simulink model "b_2x_8a_r308d"  (Simulink 6.2)
settings: Solver=ode45  StartTime=0.0  StopTime=1030.0  RelTol=1e-3
undefined symbols (not defined in the file): ant_bits, BEE2_usr, blockCountBits, blockRowBits, cmult_4bit_em
libraries: xbsIndex_r3 x3300, xps_library x102, casper_library x97
(part 1 of 22)
settings Model: LastModifiedBy=manley
settings DebuggingCC: SolverPrmCheckMsg=warning

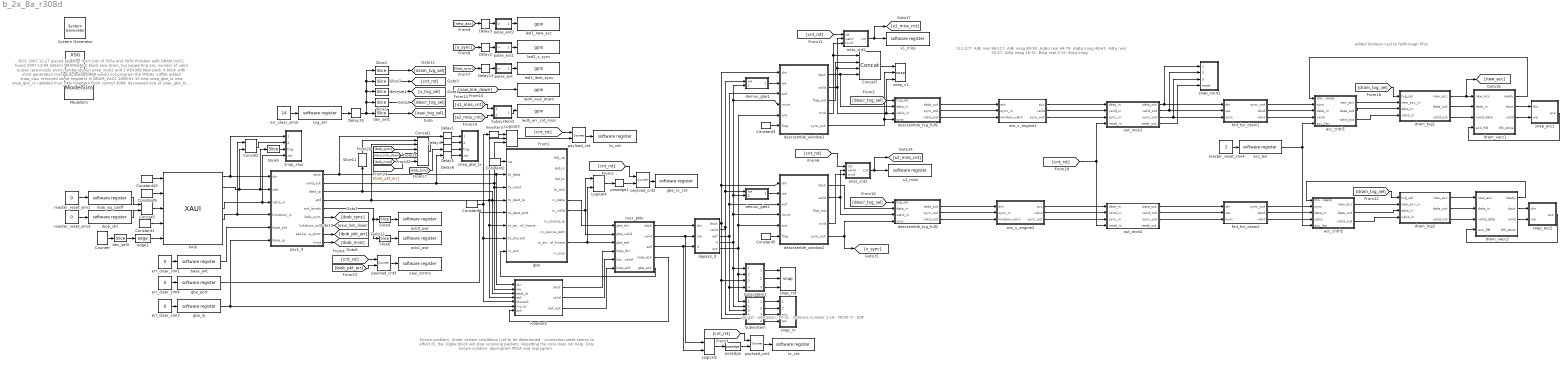
== system b_2x_8a_r308d ==
  note: 307c 2007-11-27
      | pieced together from bits of 307a and 307b
      | Problem with DRAM VACC found
      | 2007-12-04
      | Interim DRAM VACC block
      | new dram_tvg supporting any number of valid pulses (previously even numbers only)
      | snap_xout1 and 2
      | REV308
      | New pack_it block with mcnt generation moved to ibob
      |
      | BORPH would not program the FPGAs
      |
      | +308c
      | added snap_xaui
      | removed some registers in DRAM_VACC
      |
      | 2008-01-15
      | new snap_gbe_tx
      | new snap_gbe_rx
      | updated mux_pkts loopback flush control
      |
      | 308d:
      | decreased size of snap_gbe_tx, snap_gbe_rx blocks and snap_xout1 to ease routing
      | added dealy blocks to snap_gbe_tx
      | 22 Jan:
      | removed snap_gbe_rx, added snap_rx
      | 24 Jan:
      | replaced descramble onwards with version from rev307f
  note: Known problem:
      | Under certain conditions (yet to be determined - connection state seems to affect it),
      | the 10gbe block will stop receiving packets. Resetting the core does not help.
      | Only known solution: deprogram FPGA and reprogram.
  note: 112-127: AiBi real
      | 96-111: AiBi imag
      | 80-95: AqBq real
      | 64-79: AqBq imag
      | 48-63: AiBq real
      | 32-47: AiBq imag
      | 16-31: BiAq real
      | 0-15: BiAq imag
  note: added boolean cast to fallthrough fifos
  note: oob bit - allocation:
      | 17-31 - Antenna number
      | 1-16 - MCNT
      | 0 - EOF
  " System Generator" : xbsIndex_r3/ System Generator  Tag=genX  xilinxfamily=Virtex2P  part=xc2vp70  speed=-7  package=ff1704  synthesis_tool=XST  directory=./b_2x_8a_r308d/sysgen  testbench=off  simulink_period=1  sysclk_period=4.878  incr_netlist=off  trim_vbits=Everywhere in SubSystem  dbl_ovrd=According to Block Masks  core_generation=According to Block Masks  run_coregen=off  deprecated_control=off  eval_field=0
      settings: AttributesFormatString=System\nGenerator
  Concat1 : xbsIndex_r3/Concat  num_inputs=6  explicit_period=off  period=1  dbl_ovrd=off
  Concat2 : xbsIndex_r3/Concat  num_inputs=2  explicit_period=off  period=1  dbl_ovrd=off
  Concat3 : xbsIndex_r3/Concat  num_inputs=2  explicit_period=off  period=1  dbl_ovrd=off
  Concat7 : xbsIndex_r3/Concat  num_inputs=4  explicit_period=off  period=1  dbl_ovrd=off
  Constant1 : xbsIndex_r3/Constant  const=0  equ=P=C  arith_type=Unsigned  n_bits=64  bin_pt=0  opselect=C  inp2=PCIN>>17  opr=+  inp1=P  carry=CIN  iostate=0  explicit_period=on  period=1  dbl_ovrd=off
  Constant10 : xbsIndex_r3/Constant  const=1  equ=P=C  arith_type=Boolean  n_bits=1  bin_pt=0  opselect=C  inp2=PCIN>>17  opr=+  inp1=P  carry=CIN  iostate=0  explicit_period=on  period=1  dbl_ovrd=off
  Constant2 : xbsIndex_r3/Constant  const=0  equ=P=C  arith_type=Boolean  n_bits=1  bin_pt=0  opselect=C  inp2=PCIN>>17  opr=+  inp1=P  carry=CIN  iostate=0  explicit_period=on  period=1  dbl_ovrd=off
  Constant3 : xbsIndex_r3/Constant  const=0  equ=P=C  arith_type=Unsigned  n_bits=1  bin_pt=0  opselect=C  inp2=PCIN>>17  opr=+  inp1=P  carry=CIN  iostate=0  explicit_period=on  period=1  dbl_ovrd=off
  Constant5 : xbsIndex_r3/Constant  const=0  equ=P=C  arith_type=Unsigned  n_bits=1  bin_pt=0  opselect=C  inp2=PCIN>>17  opr=+  inp1=P  carry=CIN  iostate=0  explicit_period=on  period=1  dbl_ovrd=off
  Constant6 : xbsIndex_r3/Constant  const=0  equ=P=C  arith_type=Boolean  n_bits=16  bin_pt=0  opselect=C  inp2=PCIN>>17  opr=+  inp1=P  carry=CIN  iostate=0  explicit_period=on  period=1  dbl_ovrd=off
  Constant9 : xbsIndex_r3/Constant  const=0  equ=P=C  arith_type=Boolean  n_bits=1  bin_pt=0  opselect=C  inp2=PCIN>>17  opr=+  inp1=P  carry=CIN  iostate=0  explicit_period=on  period=1  dbl_ovrd=off
  Counter : xbsIndex_r3/Counter  cnt_type=Free Running  n_bits=4  bin_pt=0  arith_type=Unsigned  start_count=0  cnt_to=Inf  cnt_by_val=1  operation=Up  explicit_period=off  period=1  load_pin=off  rst=off  en=off  dbl_ovrd=off  show_param=off  use_rpm=on  gen_core=off
      settings: xl_area=[0, 0, 0, 0, 0, 0, 0]
  Delay{1,4..6,19} (5 alike) : xbsIndex_r3/Delay  latency=2  reg_retiming=on  explicit_period=off  period=1  en=off  accept_only_valid=off  init_zero=on  dbl_ovrd=off  show_param=off
      settings: xl_area=[0, 0, 0, 0, 0, 0, 0]
  Delay13 : xbsIndex_r3/Delay  latency=1  reg_retiming=on  explicit_period=off  period=1  en=off  accept_only_valid=off  init_zero=on  dbl_ovrd=off  show_param=off
      settings: xl_area=[0, 0, 0, 0, 0, 0, 0]
  Delay2 : xbsIndex_r3/Delay  latency=1  reg_retiming=on  explicit_period=off  period=1  en=off  accept_only_valid=off  init_zero=on  dbl_ovrd=off  show_param=off
      settings: xl_area=[0, 0, 0, 0, 0, 0, 0]
  Delay3 : xbsIndex_r3/Delay  latency=1  reg_retiming=on  explicit_period=off  period=1  en=off  accept_only_valid=off  init_zero=on  dbl_ovrd=off  show_param=off
      settings: xl_area=[0, 0, 0, 0, 0, 0, 0]
  Inverter3 : xbsIndex_r3/Inverter  latency=0  explicit_period=off  period=1  en=off  dbl_ovrd=off  show_param=off
      settings: xl_area=[0, 0, 0, 0, 0, 0, 0]
  Logical2 : xbsIndex_r3/Logical  logical_function=AND  inputs=2  precision=Full  arith_type=Unsigned  n_bits=8  bin_pt=2  align_bp=on  latency=0  explicit_period=on  period=1  en=off  dbl_ovrd=off  show_param=off
      settings: xl_area=[0, 0, 0, 0, 0, 0, 0]
  Logical3 : xbsIndex_r3/Logical  logical_function=AND  inputs=3  precision=Full  arith_type=Unsigned  n_bits=8  bin_pt=2  align_bp=on  latency=0  explicit_period=on  period=1  en=off  dbl_ovrd=off  show_param=off
      settings: xl_area=[0, 0, 0, 0, 0, 0, 0]
  Logical4 : xbsIndex_r3/Logical  logical_function=AND  inputs=2  precision=Full  arith_type=Unsigned  n_bits=8  bin_pt=2  align_bp=on  latency=0  explicit_period=on  period=1  en=off  dbl_ovrd=off  show_param=off
      settings: xl_area=[0, 0, 0, 0, 0, 0, 0]
  ModelSim : xbsIndex_r3/ModelSim  dir=./modelsim  waveform=on  leave_open=on  skip_compile=off  custom_scripts=off  startup_timeout=40
  Slice1 : xbsIndex_r3/Slice  mode=Lower Bit Location + Width  nbits=2  bit1=0  base1=MSB of Input  bit0=1  base0=LSB of Input  boolean_output=off  explicit_period=off  period=1  dbl_ovrd=off
  Slice11 : xbsIndex_r3/Slice  Orientation=up  mode=Lower Bit Location + Width  nbits=24  bit1=0  base1=MSB of Input  bit0=0  base0=LSB of Input  boolean_output=on  explicit_period=off  period=1  dbl_ovrd=off
  Slice2 : xbsIndex_r3/Slice  mode=Lower Bit Location + Width  nbits=6  bit1=0  base1=MSB of Input  bit0=9  base0=LSB of Input  boolean_output=off  explicit_period=off  period=1  dbl_ovrd=off
  Slice4 : xbsIndex_r3/Slice  mode=Lower Bit Location + Width  nbits=32  bit1=0  base1=MSB of Input  bit0=32  base0=LSB of Input  boolean_output=off  explicit_period=off  period=1  dbl_ovrd=off
  Slice6 : xbsIndex_r3/Slice  mode=Lower Bit Location + Width  nbits=32  bit1=0  base1=MSB of Input  bit0=0  base0=LSB of Input  boolean_output=off  explicit_period=off  period=1  dbl_ovrd=off
  Slice7 : xbsIndex_r3/Slice  mode=Lower Bit Location + Width  nbits=1  bit1=0  base1=MSB of Input  bit0=8  base0=LSB of Input  boolean_output=on  explicit_period=off  period=1  dbl_ovrd=off
  Slice9 : xbsIndex_r3/Slice  mode=Lower Bit Location + Width  nbits=1  bit1=0  base1=MSB of Input  bit0=1  base0=LSB of Input  boolean_output=on  explicit_period=off  period=1  dbl_ovrd=off
  Subsystem : Subsystem
  Subsystem1 : Subsystem
  Subsystem2 : Subsystem
  XAUI : xps_library/XAUI  Tag=xps:xaui  demux=1  port=BEE2_usr:0  show_param=off  pre_emph=3  swing=800
  XSG core config : xps_library/XSG core config  Tag=xps:xsg  hw_sys=BEE2_usr  ibob_linux=off  clk_src=sys_clk2x  gpio_clk_io_group=iBOB:sma  gpio_clk_bit_index=0  clk_rate=205  sample_period=1  synthesis_tool=XST  mpc_type=powerpc405
  acc_cntrl1 : Subsystem
  acc_cntrl2 : Subsystem
  acc_len : xps_library/software register  Tag=xps:sw_reg  io_dir=From Processor  arith_type=Unsigned  bitwidth=32  bin_pt=0  sample_period=1  gw_name=b_2x_8a_r308d_acc_len_user_data_out
  adc0_pwr : xps_library/software register  Tag=xps:sw_reg  io_dir=To Processor  arith_type=Unsigned  bitwidth=32  bin_pt=0  sample_period=1  gw_name=b_2x_8a_r308d_adc0_pwr_user_data_in
  adc1_pwr : xps_library/software register  Tag=xps:sw_reg  io_dir=To Processor  arith_type=Unsigned  bitwidth=32  bin_pt=0  sample_period=1  gw_name=b_2x_8a_r308d_adc1_pwr_user_data_in
  base_ant : xps_library/software register  Tag=xps:sw_reg  io_dir=From Processor  arith_type=Unsigned  bitwidth=32  bin_pt=0  sample_period=1  gw_name=b_2x_8a_r308d_base_ant_user_data_out
  demux_gbe1 : Subsystem  mask{share_bits=1, nx=0}
      mask prompts: share_bits "Number of X engines per GbE link (2^?)"; nx "This is X engine (? < # above) for this GbE link"
  demux_gbe2 : Subsystem  mask{share_bits=1, nx=1}
      mask prompts: share_bits "Number of X engines per GbE link (2^?)"; nx "This is X engine (? < # above) for this GbE link"
  depack_it : Subsystem  mask{payload_len=32}
      mask prompts: payload_len "Payload Length"
      mask init:
      | payload_bits = ceil(log2(payload_len));
      | packet_len = payload_len + 1;
      | packet_bits = ceil(log2(packet_len));
  descramble_tvg_full1 : Subsystem  mask{ant_bits=3, x_int_bits=7, sync_period=18}
      mask prompts: ant_bits "Number of Antennas (2^?):"; x_int_bits "X Integration Length (2^?):"; sync_period "Sync Pulse Period (2^?):"
  descramble_tvg_full2 : Subsystem  mask{ant_bits=3, x_int_bits=7, sync_period=18}
      mask prompts: ant_bits "Number of Antennas (2^?):"; x_int_bits "X Integration Length (2^?):"; sync_period "Sync Pulse Period (2^?):"
  descramble_window1 : Subsystem  mask{ant_bits=3, x_int_bits=7, window_bits=3, sync_bits=18}
      mask prompts: ant_bits "Maximum Number of Antennas (2^?):"; x_int_bits "X Engine Integration Length (2^?):"; window_bits "Number of Windows to Buffer (2^?):"; sync_bits "Samples Between Sync Pulses (2^?)"
  descramble_window2 : Subsystem  mask{ant_bits=3, x_int_bits=7, window_bits=3, sync_bits=18}
      mask prompts: ant_bits "Maximum Number of Antennas (2^?):"; x_int_bits "X Engine Integration Length (2^?):"; window_bits "Number of Windows to Buffer (2^?):"; sync_bits "Samples Between Sync Pulses (2^?)"
  dev_sel1 : xbsIndex_r3/Slice  mode=Lower Bit Location + Width  nbits=1  bit1=0  base1=MSB of Input  bit0=0  base0=LSB of Input  boolean_output=off  explicit_period=off  period=1  dbl_ovrd=off
  dev_sel3 : xbsIndex_r3/Slice  mode=Lower Bit Location + Width  nbits=1  bit1=0  base1=MSB of Input  bit0=3  base0=LSB of Input  boolean_output=on  explicit_period=off  period=1  dbl_ovrd=off
  dev_sel4 : xbsIndex_r3/Slice  mode=Lower Bit Location + Width  nbits=2  bit1=0  base1=MSB of Input  bit0=3  base0=LSB of Input  boolean_output=off  explicit_period=off  period=1  dbl_ovrd=off
  dram_tvg1 : Subsystem  mask{len=18432}
      mask prompts: len "Number of Vectors"
      mask init:
      | fmtstr = sprintf('Vector Length: %d', len);
      | set_param(gcb, 'AttributesFormatString', fmtstr);
      settings: AttributesFormatString=Vector Length: 18432
  dram_tvg2 : Subsystem  mask{len=18432}
      mask prompts: len "Number of Vectors"
      mask init:
      | fmtstr = sprintf('Vector Length: %d', len);
      | set_param(gcb, 'AttributesFormatString', fmtstr);
      settings: AttributesFormatString=Vector Length: 18432
  dram_vacc1 : Subsystem  mask{acc_length=18432}
      mask prompts: acc_length "Vector length??(# cycles)"
      mask init:
      | valid_length = 36;
  dram_vacc2 : Subsystem  mask{acc_length=18432}
      mask prompts: acc_length "Vector length??(# cycles)"
      mask init:
      | valid_length = 36;
  edge1 : casper_library/Misc/edge
  err_clear_sim1 : Constant  Value=0
  err_clear_sim3 : Constant  Value=0
  err_clear_sim4 : Constant  Value=0
  err_clear_sim5 : Constant  Value=24
  fmt_for_dram1 : Subsystem  mask{x_int_bits=7, x_n_bits=4}
      mask prompts: x_int_bits "X Engine integration length (2^?):"; x_n_bits "X Engine input bits"
  fmt_for_dram2 : Subsystem  mask{x_int_bits=7, x_n_bits=4}
      mask prompts: x_int_bits "X Engine integration length (2^?):"; x_n_bits "X Engine input bits"
  gbe : Subsystem  Tag=xps:tengbe  AncestorBlock=xps_library/ten_GbE  mask{port=BEE2_usr:2, mac_lite=on, show_param=off, pre_emph=3, swing=800}
      mask prompts: mac_lite "Use light-weight MAC: Warning --> it DOES NOT check any CRC on receive"; show_param "---------------------- Show Implementation Parameters -----------------------------------------------------------------------------------"; pre_emph "Pre-emphasis"; swing "Differential swing"
      mask init:
      | tengbe_mask;
      mask StyleString: popup(iBOB:0|iBOB:1|BEE2_ctrl:0|BEE2_ctrl:1|BEE2_usr:0|BEE2_usr:1|BEE2_usr:2|BEE2_usr:3|CORR:0),checkbox,checkbox,popup(0|1|2|3),popup(400|500|600|700|800)
      mask CallbackString:
      | ||myname=gcb;
      | if strcmp(get_param(myname, 'show_param'), 'on')
      |     set_param(myname, 'MaskVisibilities', {'on','on','on','on', 'on'});
      | else
      |     set_param(myname, 'MaskVisibilities', {'on','on','on','off','off'});
      | end||
  gbe_ip : xps_library/software register  Tag=xps:sw_reg  io_dir=From Processor  arith_type=Unsigned  bitwidth=32  bin_pt=0  sample_period=1  gw_name=b_2x_8a_r308d_gbe_ip_user_data_out
  gbe_port : xps_library/software register  Tag=xps:sw_reg  io_dir=From Processor  arith_type=Unsigned  bitwidth=32  bin_pt=0  sample_period=1  gw_name=b_2x_8a_r308d_gbe_port_user_data_out
  gbe_rx_cnt : xps_library/software register  Tag=xps:sw_reg  io_dir=To Processor  arith_type=Unsigned  bitwidth=32  bin_pt=0  sample_period=1  gw_name=b_2x_8a_r308d_gbe_rx_cnt_user_data_in
  ibob_ctrl : xps_library/software register  Tag=xps:sw_reg  io_dir=From Processor  arith_type=Unsigned  bitwidth=32  bin_pt=0  sample_period=1  gw_name=b_2x_8a_r308d_ibob_ctrl_user_data_out
  ibob_eq_coeff : xps_library/software register  Tag=xps:sw_reg  io_dir=From Processor  arith_type=Unsigned  bitwidth=32  bin_pt=0  sample_period=1  gw_name=b_2x_8a_r308d_ibob_eq_coeff_user_data_out
  led1_new_acc : xps_library/gpio  Tag=xps:gpio  io_group=BEE2_usr:led  io_dir=out  arith_type=Boolean  bitwidth=1  bin_pt=0  bit_index=0  sample_period=1  use_single_ended=off  use_ddr=off  reg_iob=off  reg_clk_phase=0  termination=None
  led2_x_sync : xps_library/gpio  Tag=xps:gpio  io_group=BEE2_usr:led  io_dir=out  arith_type=Boolean  bitwidth=1  bin_pt=0  bit_index=1  sample_period=1  use_single_ended=off  use_ddr=off  reg_iob=off  reg_clk_phase=0  termination=None
  led3_ibob_sync : xps_library/gpio  Tag=xps:gpio  io_group=BEE2_usr:led  io_dir=out  arith_type=Boolean  bitwidth=1  bin_pt=0  bit_index=2  sample_period=1  use_single_ended=off  use_ddr=off  reg_iob=off  reg_clk_phase=0  termination=None
  led4_xaui_down : xps_library/gpio  Tag=xps:gpio  io_group=BEE2_usr:led  io_dir=out  arith_type=Boolean  bitwidth=1  bin_pt=0  bit_index=3  sample_period=1  use_single_ended=off  use_ddr=off  reg_iob=off  reg_clk_phase=0  termination=None
  led5_err_cnt_miss : xps_library/gpio  Tag=xps:gpio  io_group=BEE2_usr:led  io_dir=out  arith_type=Boolean  bitwidth=1  bin_pt=0  bit_index=4  sample_period=1  use_single_ended=off  use_ddr=off  reg_iob=off  reg_clk_phase=0  termination=None
  loopback : Subsystem  mask{depth_bits=8}
      mask prompts: depth_bits "Buffer Size (2^?):"
      mask help: A loopback is a buffer for holding packets which are to be transmitted to one's self. Most switches drop any packets which have a destination IP address equal to the address of the transmitter. Thus, a seperate buffer is needed to collect these packets for readback.
  master_reset_sim1 : Constant  Value=0
  master_reset_sim3 : Constant  Value=0
  master_reset_sim4 : Constant  Value=2
  miss_cnt1 : Subsystem
  miss_cnt2 : Subsystem
  mux_pkts : Subsystem
  out_mon1 : Subsystem  mask{n_ants=8, n_chans=2048}
      mask prompts: n_ants "Number of Antennas"; n_chans "Number of Frequency Channels in the system"
  out_mon2 : Subsystem  mask{n_ants=8, n_chans=2048}
      mask prompts: n_ants "Number of Antennas"; n_chans "Number of Frequency Channels in the system"
  pack_it : Subsystem  mask{payload_len=32, ant_bits=3, skip_bits=1}
      mask prompts: payload_len "Payload Length (in 64 bit words)"; ant_bits "Number of Antennas (2^?)"; skip_bits "X engines per IP address"
      mask help: Packetizes data coming in over a XAUI interface. A packet consists of a 64 bit header (48 bits of "mcnt" and 16 bits of antenna), followed by 64 x "payload" bits of payload. "Mcnt" (master count) is a counter which keeps track of how many packets have been transmitted since the last "mrst".
      mask init:
      | packet_len = payload_len + 1;
      | packet_bits = ceil(log2(packet_len));
      | payload_bits = ceil(log2(payload_len));
  payload_cnt : xbsIndex_r3/Counter  cnt_type=Free Running  n_bits=32  bin_pt=0  arith_type=Unsigned  start_count=0  cnt_to=0  cnt_by_val=1  operation=Up  explicit_period=off  period=1  load_pin=off  rst=on  en=on  dbl_ovrd=off  show_param=off  use_rpm=on  gen_core=off
      settings: xl_area=[0, 0, 0, 0, 0, 0, 0]
  payload_cnt1 : xbsIndex_r3/Counter  cnt_type=Free Running  n_bits=32  bin_pt=0  arith_type=Unsigned  start_count=0  cnt_to=0  cnt_by_val=1  operation=Up  explicit_period=on  period=1  load_pin=off  rst=on  en=on  dbl_ovrd=off  show_param=off  use_rpm=on  gen_core=off
      settings: xl_area=[0, 0, 0, 0, 0, 0, 0]
  payload_cnt2 : xbsIndex_r3/Counter  cnt_type=Free Running  n_bits=32  bin_pt=0  arith_type=Unsigned  start_count=0  cnt_to=0  cnt_by_val=1  operation=Up  explicit_period=on  period=1  load_pin=off  rst=on  en=on  dbl_ovrd=off  show_param=off  use_rpm=on  gen_core=off
      settings: xl_area=[0, 0, 0, 0, 0, 0, 0]
  payload_cnt3 : xbsIndex_r3/Counter  cnt_type=Free Running  n_bits=32  bin_pt=0  arith_type=Unsigned  start_count=0  cnt_to=0  cnt_by_val=1  operation=Up  explicit_period=off  period=1  load_pin=off  rst=on  en=on  dbl_ovrd=off  show_param=off  use_rpm=on  gen_core=off
      settings: xl_area=[0, 0, 0, 0, 0, 0, 0]
  posedge : casper_library/Misc/posedge  Tag=Rising Edge Detector
  posedge1 : casper_library/Misc/posedge  Tag=Rising Edge Detector
  pulse_ext : Subsystem  mask{pulse_len=2^23}
      mask prompts: pulse_len "Length of Pulse"
      mask init:
      | bits = ceil(log2(pulse_len));
  pulse_ext1 : Subsystem  mask{pulse_len=2^23}
      mask prompts: pulse_len "Length of Pulse"
      mask init:
      | bits = ceil(log2(pulse_len));
  pulse_ext2 : Subsystem  mask{pulse_len=2^23}
      mask prompts: pulse_len "Length of Pulse"
      mask init:
      | bits = ceil(log2(pulse_len));
  rx_cnt : xps_library/software register  Tag=xps:sw_reg  io_dir=To Processor  arith_type=Unsigned  bitwidth=32  bin_pt=0  sample_period=1  gw_name=b_2x_8a_r308d_rx_cnt_user_data_in
  snap_acc1 : Subsystem
  snap_acc2 : Subsystem
  snap_cnt : casper_library/Scopes/snap  nsamples=11
  snap_gbe_tx : Subsystem  AncestorBlock=casper_library/Scopes/snap64  mask(snap64){nsamples=11}
      mask prompts: nsamples "No. of samples(2^?)"
      mask help:
      | The <i>snap</i> block provides a packaged solution to capturing data from
      | the FPGA fabric and making it accessible from the CPU.  The block comes in
      | 2 flavors: <i>snap</i> (which captures to a 32 bit wide Shared BRAM), and
      | <i>snap64</i> (which captures to 2x32 bit wide Shared BRAMs to effect a
      | 64 bit capture).
      mask Help: eval('xlWeb([getenv(''MLIB_ROOT''), ''\casper_library\doc\snap_usage.html''])')
  snap_rx : Subsystem  AncestorBlock=casper_library/Scopes/snap64  mask(snap64){nsamples=11}
      mask prompts: nsamples "No. of samples(2^?)"
      mask help:
      | The <i>snap</i> block provides a packaged solution to capturing data from
      | the FPGA fabric and making it accessible from the CPU.  The block comes in
      | 2 flavors: <i>snap</i> (which captures to a 32 bit wide Shared BRAM), and
      | <i>snap64</i> (which captures to 2x32 bit wide Shared BRAMs to effect a
      | 64 bit capture).
      mask Help: eval('xlWeb([getenv(''MLIB_ROOT''), ''\casper_library\doc\snap_usage.html''])')
  snap_x1 : casper_library/Scopes/snap  nsamples=12
  snap_xaui : Subsystem  AncestorBlock=casper_library/Scopes/snap64  mask(snap64){nsamples=12}
      mask prompts: nsamples "No. of samples(2^?)"
      mask help:
      | The <i>snap</i> block provides a packaged solution to capturing data from
      | the FPGA fabric and making it accessible from the CPU.  The block comes in
      | 2 flavors: <i>snap</i> (which captures to a 32 bit wide Shared BRAM), and
      | <i>snap64</i> (which captures to 2x32 bit wide Shared BRAMs to effect a
      | 64 bit capture).
      mask Help: eval('xlWeb([getenv(''MLIB_ROOT''), ''\casper_library\doc\snap_usage.html''])')
  snap_xout1 : Subsystem
  tvg_sel : xps_library/software register  Tag=xps:sw_reg  io_dir=From Processor  arith_type=Unsigned  bitwidth=32  bin_pt=0  sample_period=1  gw_name=b_2x_8a_r308d_tvg_sel_user_data_out
  tx_cnt : xps_library/software register  Tag=xps:sw_reg  io_dir=To Processor  arith_type=Unsigned  bitwidth=32  bin_pt=0  sample_period=1  gw_name=b_2x_8a_r308d_tx_cnt_user_data_in
  win_x_engine1 : Subsystem  AncestorBlock=casper_library/Correlator/x_engine  mask(x_engine){n_ants=8, n_bits=4, acc_len=128, add_latency=1, mult_latency=1, bram_latency=1, use_ded_mult=1, use_bram_delay=1}
      mask prompts: n_ants "Number of Antennas"; n_bits "Bit Width of Samples In"; acc_len "Accumulation Length"; add_latency "Add Latency"; mult_latency "Mult Latency"; bram_latency "BRAM Latency"; use_ded_mult "Multiplier Type (0=slices 1=embedded 2=bram)"; use_bram_delay "Delay in BRAM"
      mask init:
      | bit_growth = ceil(log2(acc_len));
      | ant_bits = ceil(log2(n_ants));
      | n_bits_out = (2*n_bits + 1 + bit_growth);
      | 
      | win_x_engine_init(gcb, ...
      |     'n_ants', n_ants, ...
      |     'n_bits', n_bits, ...
      |     'acc_len', acc_len, ...
      |     'add_latency', add_latency, ...
      |     'mult_latency', mult_latency, ...
      |     'bram_latency', bram_latency, ...
      |     'use_ded_mult', use_ded_mult, ...
      |     'use_bram_delay', use_bram_delay);
      settings: AttributesFormatString=n_ant=8, bits=4, mult=1, bram=1
  win_x_engine2 : Subsystem  AncestorBlock=casper_library/Correlator/x_engine  mask(x_engine){n_ants=8, n_bits=4, acc_len=128, add_latency=1, mult_latency=1, bram_latency=1, use_ded_mult=1, use_bram_delay=1}
      mask prompts: n_ants "Number of Antennas"; n_bits "Bit Width of Samples In"; acc_len "Accumulation Length"; add_latency "Add Latency"; mult_latency "Mult Latency"; bram_latency "BRAM Latency"; use_ded_mult "Multiplier Type (0=slices 1=embedded 2=bram)"; use_bram_delay "Delay in BRAM"
      mask init: same as b_2x_8a_r308d/win_x_engine1
      settings: AttributesFormatString=n_ant=8, bits=4, mult=1, bram=1
  x1_miss : xps_library/software register  Tag=xps:sw_reg  io_dir=To Processor  arith_type=Unsigned  bitwidth=32  bin_pt=0  sample_period=1  gw_name=b_2x_8a_r308d_x1_miss_user_data_in
  x2_miss : xps_library/software register  Tag=xps:sw_reg  io_dir=To Processor  arith_type=Unsigned  bitwidth=32  bin_pt=0  sample_period=1  gw_name=b_2x_8a_r308d_x2_miss_user_data_in
  xaui_errors : xps_library/software register  Tag=xps:sw_reg  io_dir=To Processor  arith_type=Unsigned  bitwidth=32  bin_pt=0  sample_period=1  gw_name=b_2x_8a_r308d_xaui_errors_user_data_in
  wires:
  err_clear_sim4/1 -> gbe_port/1
  gbe_port/1 -> gbe/5(tx_dest_port)
  err_clear_sim1/1 -> base_ant/1
  Constant2/1 -> gbe/1(rst)
  gbe/9(rx_end_of_frame) -> Logical4/2, mux_pkts/3(gbe_eof)
  err_clear_sim3/1 -> gbe_ip/1
  gbe_ip/1 -> loopback/6(my_ip), pack_it/6(base_ip)
  mux_pkts/1(dout) -> depack_it/1(din)
  mux_pkts/2(valid) -> Logical2/1, depack_it/2(we)
  mux_pkts/3(eof) -> Logical2/2, depack_it/3(eof_in)
  gbe/5(rx_data) -> mux_pkts/1(gbe_din)
  loopback/1(dout) -> mux_pkts/4(loop_din)
  loopback/2(valid) -> mux_pkts/5(loop_valid)
  loopback/3(eof_out) -> mux_pkts/6(loop_eof)
  mux_pkts/4(loop_ack) -> loopback/7(ack)
  err_clear_sim5/1 -> tvg_sel/1
  tvg_sel/1 -> Delay19/1
  Delay19/1 -> dev_sel1/1, Slice1/1, dev_sel4/1, Slice2/1, Slice7/1
  dev_sel1/1 -> [xaui_tvg_sel]
  Slice1/1 -> [descr_tvg_sel]
  dev_sel4/1 -> [x_tvg_sel]
  Slice7/1 -> [cnt_rst]
  Constant6/1 -> gbe/7(tx_discard), loopback/5(discard), Inverter3/1
  gbe/6(rx_valid) -> Logical4/1, mux_pkts/2(gbe_valid)
  mux_pkts/5(gbe_ack) -> gbe/8(rx_ack)
  Inverter3/1 -> Logical3/1
  payload_cnt/1 -> tx_cnt/1
  payload_cnt2/1 -> gbe_rx_cnt/1
  Logical4/1 -> posedge1/1
  Logical3/1 -> payload_cnt/2
  [cnt_rst] -> payload_cnt/1
  posedge1/1 -> payload_cnt2/2
  [cnt_rst] -> payload_cnt2/1
  pulse_ext/1(out) -> led3_ibob_sync/1
  Delay13/1 -> pulse_ext/1(in)
  [ibob_sync] -> Delay13/1
  pulse_ext1/1(out) -> led2_x_sync/1
  Delay2/1 -> pulse_ext1/1(in)
  [x_sync] -> Delay2/1
  [x1_miss_cnt] -> Subsystem2/1(In1)
  [x2_miss_cnt] -> Subsystem2/2(In2)
  Subsystem2/1(Out1) -> led5_err_cnt_miss/1
  [xaui_link_down] -> led4_xaui_down/1
  Slice2/1 -> [dram_tvg_sel]
  pulse_ext2/1(out) -> led1_new_acc/1
  Delay3/1 -> pulse_ext2/1(in)
  [new_acc] -> Delay3/1
  Slice4/1 -> adc0_pwr/1
  Slice6/1 -> adc1_pwr/1
  [cnt_rst] -> payload_cnt3/1
  payload_cnt3/1 -> xaui_errors/1
  pack_it/1(dout) -> gbe/2(tx_data), loopback/1(din), Delay1/1
  pack_it/2(valid_out) -> gbe/3(tx_valid), loopback/2(we), Logical3/3, Delay6/1
  pack_it/3(dest_ip) -> gbe/4(tx_dest_ip), loopback/3(dest_ip), Slice11/1
  pack_it/4(eof) -> gbe/6(tx_end_of_frame), loopback/4(eof), Logical3/2, Concat1/2
  XAUI/1 -> pack_it/1(din), snap_xaui/1(data_in)
  XAUI/4 -> pack_it/3(valid_in), snap_xaui/4(we)
  XAUI/5 -> pack_it/4(linkdown_in), Concat2/1
  base_ant/1 -> pack_it/5(base_ant)
  pack_it/6(ibob_sync) -> [ibob_sync]
  pack_it/7(linkdown_out) -> [xaui_link_down]
  pack_it/5(ant_levels) -> Slice4/1, Slice6/1
  Counter/1 -> dev_sel3/1
  dev_sel3/1 -> edge1/1
  master_reset_sim3/1 -> ibob_ctrl/1
  master_reset_sim1/1 -> ibob_eq_coeff/1
  ibob_ctrl/1 -> Concat3/2
  ibob_eq_coeff/1 -> Concat3/1
  Constant10/1 -> XAUI/1
  Constant9/1 -> XAUI/2
  Concat3/1 -> XAUI/3
  Constant1/1 -> XAUI/4
  edge1/1 -> XAUI/5
  Slice9/1 -> snap_xaui/3(trig)
  Concat2/1 -> snap_xaui/2(oob_in)
  XAUI/2 -> Concat2/2, pack_it/2(oob), Slice9/1
  Concat1/1 -> Delay4/1
  Slice11/1 -> Concat1/1
  [ibob_sync] -> Delay5/1
  [ibob_sync] -> Concat1/3
  [xaui_link_down] -> Concat1/4
  pack_it/9(mrst) -> [ibob_mrst]
  [ibob_mrst] -> Concat1/5
  pack_it/8(packet_size_error) -> [ibob_pkt_err]
  [ibob_pkt_err] -> payload_cnt3/2
  [ibob_pkt_err] -> Concat1/6
  Delay1/1 -> snap_gbe_tx/1(data_in)
  Delay4/1 -> snap_gbe_tx/2(oob_in)
  Delay5/1 -> snap_gbe_tx/3(trig)
  Delay6/1 -> snap_gbe_tx/4(we)
  depack_it/2(valid) -> demux_gbe2/1(we), demux_gbe1/1(we), Subsystem/4(In6)
  Subsystem1/2(Out2) -> snap_cnt/2
  depack_it/4(mcnt) -> demux_gbe2/2(mcnt), demux_gbe1/2(mcnt), descramble_window1/4(mcnt), descramble_window2/4(mcnt), Subsystem/2(In3), Subsystem1/1(In1)
  depack_it/1(dout) -> descramble_window2/1(din), descramble_window1/1(din), Subsystem/5(In1), Subsystem1/3(In3)
  depack_it/3(eof) -> descramble_window2/3(eof), descramble_window1/3(eof), Subsystem1/4(In4), Subsystem/3(In4)
  depack_it/5(ant) -> descramble_window2/5(ant), descramble_window1/5(ant), Subsystem/1(In2), Subsystem1/2(In2)
  demux_gbe1/1(valid) -> descramble_window1/2(we)
  demux_gbe2/1(valid) -> descramble_window2/2(we)
  Subsystem1/1(Out1) -> snap_cnt/1
  Constant5/1 -> descramble_window2/6(flag)
  payload_cnt1/1 -> rx_cnt/1
  Logical2/1 -> posedge/1
  posedge/1 -> payload_cnt1/2
  [cnt_rst] -> payload_cnt1/1
  Constant3/1 -> descramble_window1/6(flag)
  descramble_window2/4(rcvd) -> miss_cnt2/3(rcvd)
  descramble_window2/2(valid) -> miss_cnt2/2(valid), descramble_tvg_full2/3(valid_in)
  descramble_window1/1(dout) -> Concat7/4, descramble_tvg_full1/2(data_in)
  descramble_window1/3(flag_out) -> Concat7/2
  descramble_window1/4(rcvd) -> Concat7/1, miss_cnt1/3(rcvd)
  descramble_window1/5(sync_out) -> snap_x1/2, descramble_tvg_full1/4(sync)
  descramble_window1/2(valid) -> Concat7/3, miss_cnt1/2(valid), snap_x1/3, descramble_tvg_full1/3(valid_in)
  miss_cnt1/1(cnt) -> x1_miss/1, [x1_miss_cnt]
  miss_cnt2/1(cnt) -> x2_miss/1, [x2_miss_cnt]
  [cnt_rst] -> miss_cnt1/1(rst)
  descramble_window2/5(sync_out) -> [x_sync], descramble_tvg_full2/4(sync)
  [cnt_rst] -> miss_cnt2/1(rst)
  [descr_tvg_sel] -> descramble_tvg_full1/1(tvg_sel)
  Concat7/1 -> snap_x1/1
  [cnt_rst] -> out_mon1/4(reset_in), out_mon2/4(reset_in)
  out_mon1/3(sync_out) -> fmt_for_dram1/3(sync), snap_xout1/3(trigger)
  out_mon1/4(reset_out) -> snap_xout1/4(reset)
  out_mon1/2(valid_out) -> fmt_for_dram1/2(we), snap_xout1/2(valid_in)
  out_mon1/1(data_out) -> fmt_for_dram1/1(din), snap_xout1/1(data_in)
  descramble_window2/1(dout) -> descramble_tvg_full2/2(data_in)
  [descr_tvg_sel] -> descramble_tvg_full2/1(tvg_sel)
  acc_len/1 -> acc_cntrl1/5(acc_len), acc_cntrl2/5(acc_len)
  master_reset_sim4/1 -> acc_len/1
  out_mon2/1(data_out) -> fmt_for_dram2/1(din)
  out_mon2/2(valid_out) -> fmt_for_dram2/2(we)
  out_mon2/3(sync_out) -> fmt_for_dram2/3(sync)
  dram_vacc1/2(dout) -> snap_acc1/1(din)
  dram_vacc1/3(valid) -> snap_acc1/2(we)
  snap_acc1/1(ack) -> dram_vacc1/4(ack_RB)
  dram_vacc2/2(dout) -> snap_acc2/1(din)
  dram_vacc2/3(valid) -> snap_acc2/2(we)
  snap_acc2/1(ack) -> dram_vacc2/4(ack_RB)
  dram_tvg1/1(new_acc) -> [new_acc], dram_vacc1/1(new_acc)
  dram_tvg1/2(data_out) -> dram_vacc1/2(data_in)
  dram_tvg1/3(valid_out) -> dram_vacc1/3(valid_data)
  dram_tvg2/1(new_acc) -> dram_vacc2/1(new_acc)
  dram_tvg2/2(data_out) -> dram_vacc2/2(data_in)
  dram_tvg2/3(valid_out) -> dram_vacc2/3(valid_data)
  [dram_tvg_sel] -> dram_tvg2/1(tvg_sel)
  [dram_tvg_sel] -> dram_tvg1/1(tvg_sel)
  fmt_for_dram1/1(sync_out) -> acc_cntrl1/2(sync)
  fmt_for_dram1/2(dout) -> acc_cntrl1/3(data_in)
  fmt_for_dram1/3(valid) -> acc_cntrl1/4("valid ")
  dram_vacc1/1(ready) -> acc_cntrl1/1(dram_ready)
  acc_cntrl1/1(new_acc) -> dram_tvg1/2(new_acc_in)
  acc_cntrl1/2(data_out) -> dram_tvg1/3(data_in)
  acc_cntrl1/3(valid_out) -> dram_tvg1/4(valid_in)
  dram_vacc2/1(ready) -> acc_cntrl2/1(dram_ready)
  acc_cntrl2/1(new_acc) -> dram_tvg2/2(new_acc_in)
  acc_cntrl2/2(data_out) -> dram_tvg2/3(data_in)
  acc_cntrl2/3(valid_out) -> dram_tvg2/4(valid_in)
  fmt_for_dram2/1(sync_out) -> acc_cntrl2/2(sync)
  fmt_for_dram2/2(dout) -> acc_cntrl2/3(data_in)
  fmt_for_dram2/3(valid) -> acc_cntrl2/4("valid ")
  descramble_tvg_full2/2(sync_out) -> win_x_engine2/2(sync_in)
  descramble_tvg_full2/3(valid_out) -> win_x_engine2/3(window_valid)
  descramble_tvg_full1/1(data_out) -> win_x_engine1/1(ant)
  descramble_tvg_full1/2(sync_out) -> win_x_engine1/2(sync_in)
  descramble_tvg_full1/3(valid_out) -> win_x_engine1/3(window_valid)
  descramble_tvg_full2/1(data_out) -> win_x_engine2/1(ant)
  win_x_engine1/1(acc) -> out_mon1/1(data_in)
  win_x_engine1/2(valid) -> out_mon1/2(valid_in)
  win_x_engine1/3(sync_out) -> out_mon1/3(sync_in)
  win_x_engine2/1(acc) -> out_mon2/1(data_in)
  win_x_engine2/2(valid) -> out_mon2/2(valid_in)
  win_x_engine2/3(sync_out) -> out_mon2/3(sync_in)
  Subsystem/1(Out1) -> snap_rx/1(data_in)
  Subsystem/2(Out2) -> snap_rx/2(oob_in)
  Subsystem/3(Out3) -> snap_rx/3(trig)
  Subsystem/4(Out4) -> snap_rx/4(we)
  Subsystem1/3(Out3) -> snap_cnt/3

== system b_2x_8a_r308d/Subsystem ==
  In2 : Inport  Port=1  LatchInput=off
  In3 : Inport  Port=2  LatchInput=off
  In4 : Inport  Port=3  LatchInput=off
  In6 : Inport  Port=4  LatchInput=off
  In1 : Inport  Port=5  LatchInput=off
  Concat4 : xbsIndex_r3/Concat  num_inputs=3  explicit_period=off  period=1  dbl_ovrd=off
  Delay{9..10,12,14} (4 alike) : xbsIndex_r3/Delay  latency=2  reg_retiming=on  explicit_period=off  period=1  en=off  accept_only_valid=off  init_zero=on  dbl_ovrd=off  show_param=off
      settings: xl_area=[0, 0, 0, 0, 0, 0, 0]
  Slice10 : xbsIndex_r3/Slice  mode=Lower Bit Location + Width  nbits=16  bit1=0  base1=MSB of Input  bit0=0  base0=LSB of Input  boolean_output=off  explicit_period=off  period=1  dbl_ovrd=off
  Slice13 : xbsIndex_r3/Slice  mode=Lower Bit Location + Width  nbits=15  bit1=0  base1=MSB of Input  bit0=0  base0=LSB of Input  boolean_output=off  explicit_period=off  period=1  dbl_ovrd=off
  Out1 : Outport
  Out2 : Outport  Port=2
  Out3 : Outport  Port=3
  Out4 : Outport  Port=4
  wires:
  Concat4/1 -> Delay14/1
  Slice10/1 -> Concat4/2
  Slice13/1 -> Concat4/1
  In1/1 -> Delay9/1
  In2/1 -> Slice13/1
  In3/1 -> Slice10/1
  In4/1 -> Concat4/3, Delay10/1
  In6/1 -> Delay12/1
  Delay9/1 -> Out1/1
  Delay14/1 -> Out2/1
  Delay10/1 -> Out3/1
  Delay12/1 -> Out4/1

== system b_2x_8a_r308d/Subsystem1 ==
  In1 : Inport  Port=1  LatchInput=off
  In2 : Inport  Port=2  LatchInput=off
  In3 : Inport  Port=3  LatchInput=off
  In4 : Inport  Port=4  LatchInput=off
  Concat9 : xbsIndex_r3/Concat  num_inputs=3  explicit_period=off  period=1  dbl_ovrd=off
  Constant15 : xbsIndex_r3/Constant  const=1  equ=P=C  arith_type=Boolean  n_bits=11  bin_pt=0  opselect=C  inp2=PCIN>>17  opr=+  inp1=P  carry=CIN  iostate=0  explicit_period=on  period=1  dbl_ovrd=off
  Slice12 : xbsIndex_r3/Slice  mode=Lower Bit Location + Width  nbits=8  bit1=0  base1=MSB of Input  bit0=0  base0=LSB of Input  boolean_output=off  explicit_period=off  period=1  dbl_ovrd=off
  Slice15 : xbsIndex_r3/Slice  mode=Lower Bit Location + Width  nbits=8  bit1=0  base1=MSB of Input  bit0=8  base0=LSB of Input  boolean_output=off  explicit_period=off  period=1  dbl_ovrd=off
  Slice8 : xbsIndex_r3/Slice  mode=Lower Bit Location + Width  nbits=16  bit1=0  base1=MSB of Input  bit0=0  base0=LSB of Input  boolean_output=off  explicit_period=off  period=1  dbl_ovrd=off
  Out1 : Outport
  Out2 : Outport  Port=2
  Out3 : Outport  Port=3
  wires:
  Slice8/1 -> Concat9/1
  Slice12/1 -> Concat9/2
  Slice15/1 -> Concat9/3
  In1/1 -> Slice8/1
  In2/1 -> Slice12/1
  In3/1 -> Slice15/1
  Concat9/1 -> Out1/1
  Constant15/1 -> Out2/1
  In4/1 -> Out3/1

== system b_2x_8a_r308d/Subsystem2 ==
  In1 : Inport  Port=1  LatchInput=off
  In2 : Inport  Port=2  LatchInput=off
  Constant7 : xbsIndex_r3/Constant  const=0  equ=P=C  arith_type=Unsigned  n_bits=16  bin_pt=0  opselect=C  inp2=PCIN>>17  opr=+  inp1=P  carry=CIN  iostate=0  explicit_period=on  period=1  dbl_ovrd=off
  Delay11 : xbsIndex_r3/Delay  latency=1  reg_retiming=on  explicit_period=off  period=1  en=off  accept_only_valid=off  init_zero=on  dbl_ovrd=off  show_param=off
      settings: xl_area=[0, 0, 0, 0, 0, 0, 0]
  Delay8 : xbsIndex_r3/Delay  latency=1  reg_retiming=on  explicit_period=off  period=1  en=off  accept_only_valid=off  init_zero=on  dbl_ovrd=off  show_param=off
      settings: xl_area=[0, 0, 0, 0, 0, 0, 0]
  Logical8 : xbsIndex_r3/Logical  logical_function=OR  inputs=2  precision=Full  arith_type=Unsigned  n_bits=8  bin_pt=2  align_bp=on  latency=0  explicit_period=on  period=1  en=off  dbl_ovrd=off  show_param=off
      settings: xl_area=[0, 0, 0, 0, 0, 0, 0]
  Relational : xbsIndex_r3/Relational  mode=a!=b  latency=1  explicit_period=off  period=1  en=off  dbl_ovrd=off  show_param=off
      settings: xl_area=[0, 0, 0, 0, 0, 0, 0]
  Out1 : Outport
  wires:
  Delay8/1 -> Logical8/1
  Delay11/1 -> Logical8/2
  Constant7/1 -> Relational/2
  Logical8/1 -> Relational/1
  In1/1 -> Delay8/1
  Relational/1 -> Out1/1
  In2/1 -> Delay11/1

== system b_2x_8a_r308d/acc_cntrl1 ==
  dram_ready : Inport  Port=1  LatchInput=off
  sync : Inport  Port=2  LatchInput=off
  data_in : Inport  Port=3  LatchInput=off
  "valid " : Inport  Port=4  LatchInput=off
  acc_len : Inport  Port=5  LatchInput=off
  Gateway Out{1..6,10..12} (9 alike) : xbsIndex_r3/Gateway Out  output_type=Double  nbits=8  bin_pt=6  arith_type=Boolean  quantization=Truncate  overflow=Wrap  hdl_port=off  timing_constraint=None  locs_specified=off  LOCs={}  needs_fixed_name=off  show_param=off
      settings: xl_area=[0, 0, 0, 0, 0, 0, 0]
  Logical6 : xbsIndex_r3/Logical  logical_function=AND  inputs=2  precision=Full  arith_type=Unsigned  n_bits=8  bin_pt=2  align_bp=on  latency=0  explicit_period=off  period=1  en=off  dbl_ovrd=off  show_param=off
      settings: xl_area=[0, 0, 0, 0, 0, 0, 0]
  Register1 : xbsIndex_r3/Register  init=0  reg_only_valid=off  explicit_period=off  period=1  rst=off  en=off  out_en=off  dbl_ovrd=off  show_param=off
      settings: xl_area=[0, 0, 0, 0, 0, 0, 0]
  Relational5 : xbsIndex_r3/Relational  mode=a=b  latency=0  explicit_period=on  period=1  en=off  dbl_ovrd=off  show_param=off
      settings: xl_area=[0, 0, 0, 0, 0, 0, 0]
  Scope1 : Scope  NumInputPorts=3
      settings: YMin=2.15512e+037~-1~-1  YMax=2.38198e+037~1~1  SaveName=ScopeData2
  Scope2 : Scope  NumInputPorts=3
      settings: YMin=0~1~0  YMax=3e+011~1~1  SaveName=ScopeData3
  Scope4 : Scope  NumInputPorts=3
      settings: YMin=2.15512e+037~-1~-1  YMax=2.38198e+037~1~1
  posedge : casper_library/Misc/posedge  Tag=Rising Edge Detector
  posedge1 : casper_library/Misc/posedge  Tag=Rising Edge Detector
  valid_cntr : xbsIndex_r3/Counter  cnt_type=Free Running  n_bits=32  bin_pt=0  arith_type=Unsigned  start_count=0  cnt_to=Inf  cnt_by_val=1  operation=Up  explicit_period=on  period=1  load_pin=off  rst=on  en=on  dbl_ovrd=off  show_param=off  use_rpm=on  gen_core=off
      settings: xl_area=[0, 0, 0, 0, 0, 0, 0]
  new_acc : Outport
  data_out : Outport  Port=2
  valid_out : Outport  Port=3
  wires:
  "valid "/1 -> Gateway Out1/1, valid_out/1, Gateway Out4/1
  sync/1 -> Logical6/1
  dram_ready/1 -> Logical6/2
  Logical6/1 -> Gateway Out12/1, posedge/1, Gateway Out2/1
  posedge/1 -> valid_cntr/2
  Relational5/1 -> posedge1/1, Gateway Out10/1, valid_cntr/1
  valid_cntr/1 -> Relational5/1, Gateway Out11/1
  acc_len/1 -> Relational5/2
  data_in/1 -> Gateway Out3/1, data_out/1, Gateway Out6/1
  Gateway Out11/1 -> Scope4/3
  Gateway Out10/1 -> Scope4/2
  Gateway Out12/1 -> Scope4/1
  Gateway Out2/1 -> Scope1/3
  Gateway Out1/1 -> Scope1/2
  Gateway Out3/1 -> Scope1/1
  Gateway Out5/1 -> Scope2/3
  Gateway Out4/1 -> Scope2/2
  Gateway Out6/1 -> Scope2/1
  posedge1/1 -> Register1/1
  Register1/1 -> new_acc/1, Gateway Out5/1

== system b_2x_8a_r308d/acc_cntrl2 ==
  dram_ready : Inport  Port=1  LatchInput=off
  sync : Inport  Port=2  LatchInput=off
  data_in : Inport  Port=3  LatchInput=off
  "valid " : Inport  Port=4  LatchInput=off
  acc_len : Inport  Port=5  LatchInput=off
  Gateway Out{1..6,10..12} (9 alike) : xbsIndex_r3/Gateway Out  output_type=Double  nbits=8  bin_pt=6  arith_type=Boolean  quantization=Truncate  overflow=Wrap  hdl_port=off  timing_constraint=None  locs_specified=off  LOCs={}  needs_fixed_name=off  show_param=off
      settings: xl_area=[0, 0, 0, 0, 0, 0, 0]
  Logical6 : xbsIndex_r3/Logical  logical_function=AND  inputs=2  precision=Full  arith_type=Unsigned  n_bits=8  bin_pt=2  align_bp=on  latency=0  explicit_period=off  period=1  en=off  dbl_ovrd=off  show_param=off
      settings: xl_area=[0, 0, 0, 0, 0, 0, 0]
  Register1 : xbsIndex_r3/Register  init=0  reg_only_valid=off  explicit_period=off  period=1  rst=off  en=off  out_en=off  dbl_ovrd=off  show_param=off
      settings: xl_area=[0, 0, 0, 0, 0, 0, 0]
  Relational5 : xbsIndex_r3/Relational  mode=a=b  latency=0  explicit_period=on  period=1  en=off  dbl_ovrd=off  show_param=off
      settings: xl_area=[0, 0, 0, 0, 0, 0, 0]
  Scope1 : Scope  NumInputPorts=3
      settings: YMin=2.15512e+037~-1~-1  YMax=2.38198e+037~1~1  SaveName=ScopeData2
  Scope2 : Scope  NumInputPorts=3
      settings: YMin=0~1~0  YMax=3e+011~1~1  SaveName=ScopeData3
  Scope4 : Scope  NumInputPorts=3
      settings: YMin=2.15512e+037~-1~-1  YMax=2.38198e+037~1~1
  posedge : casper_library/Misc/posedge  Tag=Rising Edge Detector
  posedge1 : casper_library/Misc/posedge  Tag=Rising Edge Detector
  valid_cntr : xbsIndex_r3/Counter  cnt_type=Free Running  n_bits=32  bin_pt=0  arith_type=Unsigned  start_count=0  cnt_to=Inf  cnt_by_val=1  operation=Up  explicit_period=on  period=1  load_pin=off  rst=on  en=on  dbl_ovrd=off  show_param=off  use_rpm=on  gen_core=off
      settings: xl_area=[0, 0, 0, 0, 0, 0, 0]
  new_acc : Outport
  data_out : Outport  Port=2
  valid_out : Outport  Port=3
  wires:
  "valid "/1 -> Gateway Out1/1, valid_out/1, Gateway Out4/1
  sync/1 -> Logical6/1
  dram_ready/1 -> Logical6/2
  Logical6/1 -> Gateway Out12/1, posedge/1, Gateway Out2/1
  posedge/1 -> valid_cntr/2
  Relational5/1 -> posedge1/1, Gateway Out10/1, valid_cntr/1
  valid_cntr/1 -> Relational5/1, Gateway Out11/1
  acc_len/1 -> Relational5/2
  data_in/1 -> Gateway Out3/1, data_out/1, Gateway Out6/1
  Gateway Out11/1 -> Scope4/3
  Gateway Out10/1 -> Scope4/2
  Gateway Out12/1 -> Scope4/1
  Gateway Out2/1 -> Scope1/3
  Gateway Out1/1 -> Scope1/2
  Gateway Out3/1 -> Scope1/1
  Gateway Out5/1 -> Scope2/3
  Gateway Out4/1 -> Scope2/2
  Gateway Out6/1 -> Scope2/1
  posedge1/1 -> Register1/1
  Register1/1 -> new_acc/1, Gateway Out5/1

== system b_2x_8a_r308d/demux_gbe1 ==
  we : Inport  Port=1  LatchInput=off
  mcnt : Inport  Port=2  LatchInput=off
  Constant1 : xbsIndex_r3/Constant  const=nx  equ=P=C  arith_type=Unsigned  n_bits=share_bits  bin_pt=0  opselect=C  inp2=PCIN>>17  opr=+  inp1=P  carry=CIN  iostate=0  explicit_period=on  period=1  dbl_ovrd=off
  Logical3 : xbsIndex_r3/Logical  logical_function=AND  inputs=2  precision=Full  arith_type=Unsigned  n_bits=8  bin_pt=2  align_bp=on  latency=0  explicit_period=on  period=1  en=off  dbl_ovrd=off  show_param=off
      settings: xl_area=[0, 0, 0, 0, 0, 0, 0]
  Relational : xbsIndex_r3/Relational  mode=a=b  latency=0  explicit_period=off  period=1  en=off  dbl_ovrd=off  show_param=off
      settings: xl_area=[0, 0, 0, 0, 0, 0, 0]
  Slice4 : xbsIndex_r3/Slice  mode=Lower Bit Location + Width  nbits=share_bits  bit1=0  base1=MSB of Input  bit0=0  base0=LSB of Input  boolean_output=off  explicit_period=off  period=1  dbl_ovrd=off
  valid : Outport
  wires:
  we/1 -> Logical3/1
  Logical3/1 -> valid/1
  mcnt/1 -> Slice4/1
  Slice4/1 -> Relational/1
  Constant1/1 -> Relational/2
  Relational/1 -> Logical3/2

== system b_2x_8a_r308d/demux_gbe2 ==
  we : Inport  Port=1  LatchInput=off
  mcnt : Inport  Port=2  LatchInput=off
  Constant1 : xbsIndex_r3/Constant  const=nx  equ=P=C  arith_type=Unsigned  n_bits=share_bits  bin_pt=0  opselect=C  inp2=PCIN>>17  opr=+  inp1=P  carry=CIN  iostate=0  explicit_period=on  period=1  dbl_ovrd=off
  Logical3 : xbsIndex_r3/Logical  logical_function=AND  inputs=2  precision=Full  arith_type=Unsigned  n_bits=8  bin_pt=2  align_bp=on  latency=0  explicit_period=on  period=1  en=off  dbl_ovrd=off  show_param=off
      settings: xl_area=[0, 0, 0, 0, 0, 0, 0]
  Relational : xbsIndex_r3/Relational  mode=a=b  latency=0  explicit_period=off  period=1  en=off  dbl_ovrd=off  show_param=off
      settings: xl_area=[0, 0, 0, 0, 0, 0, 0]
  Slice4 : xbsIndex_r3/Slice  mode=Lower Bit Location + Width  nbits=share_bits  bit1=0  base1=MSB of Input  bit0=0  base0=LSB of Input  boolean_output=off  explicit_period=off  period=1  dbl_ovrd=off
  valid : Outport
  wires:
  Relational/1 -> Logical3/2
  Constant1/1 -> Relational/2
  Slice4/1 -> Relational/1
  mcnt/1 -> Slice4/1
  Logical3/1 -> valid/1
  we/1 -> Logical3/1

== system b_2x_8a_r308d/depack_it ==
  note: The first 64 bit word in a packet
      | is 48 bits of mcnt + 16 bits of antenna.
      | This circuit counts through each
      | packet, registers mcnt and ant,
      | and presents them aligned with the
      | data packet.
  din : Inport  Port=1  LatchInput=off
  we : Inport  Port=2  LatchInput=off
  eof_in : Inport  Port=3  LatchInput=off
  Constant1 : xbsIndex_r3/Constant  const=0  equ=P=C  arith_type=Unsigned  n_bits=packet_bits  bin_pt=0  opselect=C  inp2=PCIN>>17  opr=+  inp1=P  carry=CIN  iostate=0  explicit_period=on  period=1  dbl_ovrd=off
  Delay4 : xbsIndex_r3/Delay  latency=1  reg_retiming=off  explicit_period=off  period=1  en=off  accept_only_valid=off  init_zero=on  dbl_ovrd=off  show_param=off
      settings: xl_area=[0, 0, 0, 0, 0, 0, 0]
  Delay5 : xbsIndex_r3/Delay  latency=1  reg_retiming=off  explicit_period=off  period=1  en=off  accept_only_valid=off  init_zero=on  dbl_ovrd=off  show_param=off
      settings: xl_area=[0, 0, 0, 0, 0, 0, 0]
  Inverter : xbsIndex_r3/Inverter  latency=0  explicit_period=off  period=1  en=off  dbl_ovrd=off  show_param=off
      settings: xl_area=[0, 0, 0, 0, 0, 0, 0]
  Logical1 : xbsIndex_r3/Logical  logical_function=AND  inputs=2  precision=Full  arith_type=Unsigned  n_bits=8  bin_pt=2  align_bp=on  latency=0  explicit_period=off  period=1  en=off  dbl_ovrd=off  show_param=off
      settings: xl_area=[0, 0, 0, 0, 0, 0, 0]
  Logical2 : xbsIndex_r3/Logical  logical_function=AND  inputs=2  precision=Full  arith_type=Unsigned  n_bits=8  bin_pt=2  align_bp=on  latency=1  explicit_period=off  period=1  en=off  dbl_ovrd=off  show_param=off
      settings: xl_area=[0, 0, 0, 0, 0, 0, 0]
  Logical3 : xbsIndex_r3/Logical  logical_function=AND  inputs=2  precision=Full  arith_type=Unsigned  n_bits=8  bin_pt=2  align_bp=on  latency=0  explicit_period=off  period=1  en=off  dbl_ovrd=off  show_param=off
      settings: xl_area=[0, 0, 0, 0, 0, 0, 0]
  Register : xbsIndex_r3/Register  init=0  reg_only_valid=off  explicit_period=off  period=1  rst=off  en=on  out_en=off  dbl_ovrd=off  show_param=off
      settings: xl_area=[0, 0, 0, 0, 0, 0, 0]
  Relational : xbsIndex_r3/Relational  mode=a=b  latency=0  explicit_period=off  period=1  en=off  dbl_ovrd=off  show_param=off
      settings: xl_area=[0, 0, 0, 0, 0, 0, 0]
  Slice1 : xbsIndex_r3/Slice  mode=Lower Bit Location + Width  nbits=48  bit1=0  base1=MSB of Input  bit0=16  base0=LSB of Input  boolean_output=off  explicit_period=off  period=1  dbl_ovrd=off
  Slice5 : xbsIndex_r3/Slice  mode=Lower Bit Location + Width  nbits=16  bit1=0  base1=MSB of Input  bit0=0  base0=LSB of Input  boolean_output=off  explicit_period=off  period=1  dbl_ovrd=off
  payload_cnt : xbsIndex_r3/Counter  cnt_type=Count Limited  n_bits=packet_bits  bin_pt=0  arith_type=Unsigned  start_count=0  cnt_to=packet_len - 1  cnt_by_val=1  operation=Up  explicit_period=off  period=1  load_pin=off  rst=on  en=on  dbl_ovrd=off  show_param=off  use_rpm=on  gen_core=off
      settings: xl_area=[0, 0, 0, 0, 0, 0, 0]
  dout : Outport
  valid : Outport  Port=2
  eof : Outport  Port=3
  mcnt : Outport  Port=4
  ant : Outport  Port=5
  wires:
  we/1 -> Logical2/1, Logical1/2, payload_cnt/2, Logical3/2
  Constant1/1 -> Relational/2
  payload_cnt/1 -> Relational/1
  Relational/1 -> Inverter/1, Logical1/1
  Logical2/1 -> valid/1
  Logical1/1 -> Register/2
  din/1 -> Delay4/1, Register/1
  Delay4/1 -> dout/1
  Delay5/1 -> eof/1
  Register/1 -> Slice5/1, Slice1/1
  Slice1/1 -> mcnt/1
  Slice5/1 -> ant/1
  Inverter/1 -> Logical2/2
  Logical3/1 -> payload_cnt/1, Delay5/1
  eof_in/1 -> Logical3/1
